simulink model "wheelvelocityslx"  (R2024b)
settings: Solver=VariableStepAuto  StartTime=0.0  StopTime=1000  RelTol=1e-3
undefined symbols (not defined in the file): DiscIntNeverNeededParam
libraries: simulink x3
settings Model: Creator=manda  LastModifiedBy=manda

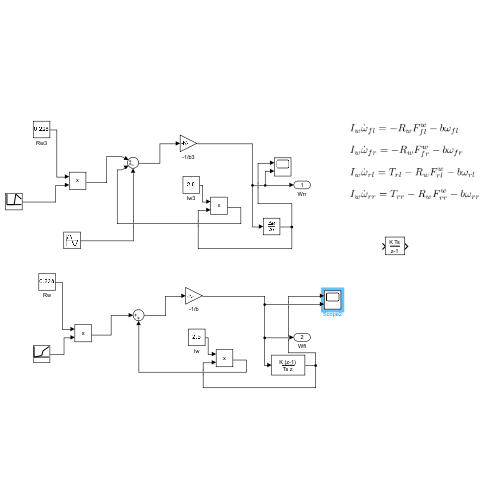
[thumbnail: Simulink's stored preview of the top-level diagram]
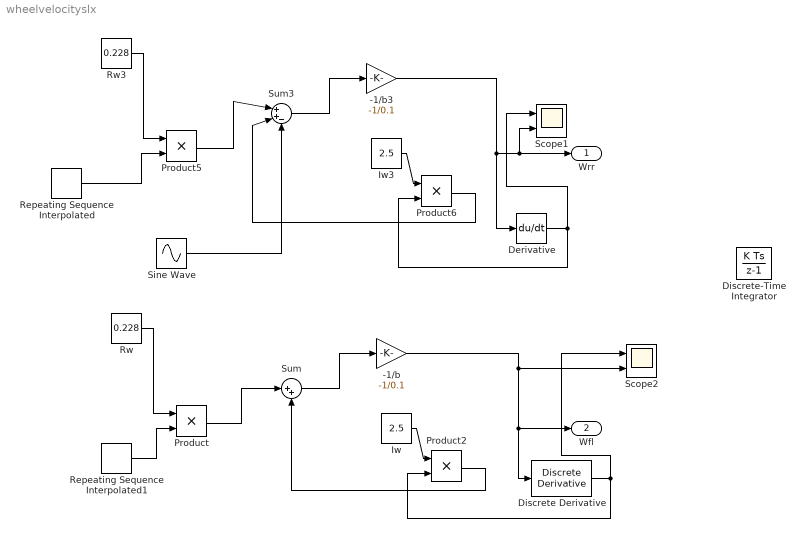
== system wheelvelocityslx ==
  -1/b : Gain  Gain=-1/0.1
  -1/b3 : Gain  Gain=-1/0.1
  Derivative : Derivative
  Discrete Derivative : simulink/Discrete/Discrete Derivative  gainval=1.0  ICPrevScaledInput=0.01  OutMin=[]  OutMax=[]  OutDataType=fixdt(1, 16)  OutScaling=2^-10  DoSatur=off
  Discrete-Time Integrator : DiscreteIntegrator  SampleTime=-1  ICPrevOutput=DiscIntNeverNeededParam  ICPrevScaledInput=DiscIntNeverNeededParam
  Iw : Constant  Value=2.5
  Iw3 : Constant  Value=2.5
  Product{,2,5..6} (4 alike) : Product
  Repeating Sequence Interpolated : simulink/Sources/Repeating Sequence Interpolated  OutValues=[0 0 0 2 1].'  TimeValues=[0 0.1 0.5 0.6 1].'  LookUpMeth=Interpolation-Use End Values  tsamp=0.01  OutMin=[]  OutMax=[]  OutDataTypeStr=double  OutputDataTypeScalingMode=double  OutDataType=fixdt(0,8)  OutScaling=2^-10
  Repeating Sequence Interpolated1 : simulink/Sources/Repeating Sequence Interpolated  OutValues=[0 0 5 20 35].'  TimeValues=[0 0.1 0.5 0.6 1].'  LookUpMeth=Interpolation-Use End Values  tsamp=0.01  OutMin=[]  OutMax=[]  OutDataTypeStr=double  OutputDataTypeScalingMode=double  OutDataType=fixdt(0,8)  OutScaling=2^-10
  Rw : Constant  Value=0.228
  Rw3 : Constant  Value=0.228
  Scope1 : Scope  NumInputPorts=2
  Scope2 : Scope  NumInputPorts=2
  Sine Wave : Sin  Amplitude=60  Phase=90  SampleTime=0
  Sum : Sum  Inputs=|++
  Sum3 : Sum  Inputs=|++-
  Wrr : Outport
  Wfl : Outport  Port=2
  wires:
  Product5/1 -> Sum3/1
  Derivative/1 -> Product6/2, Scope1/1
  -1/b3/1 -> Derivative/1, Scope1/2, Wrr/1
  Repeating Sequence Interpolated/1 -> Product5/2
  Iw3/1 -> Product6/1
  Product6/1 -> Sum3/2
  Rw3/1 -> Product5/1
  Sine Wave/1 -> Sum3/3
  Sum3/1 -> -1/b3/1
  Product2/1 -> Sum/2
  Rw/1 -> Product/1
  Product/1 -> Sum/1
  Iw/1 -> Product2/1
  Repeating Sequence Interpolated1/1 -> Product/2
  Sum/1 -> -1/b/1
  Discrete Derivative/1 -> Product2/2, Scope2/1
  -1/b/1 -> Discrete Derivative/1, Wfl/1, Scope2/2
